simulink model "MOD_TC"  (R2012b)
settings: Solver=ode45  SolverMode=SingleTasking  StartTime=0.0  StopTime=10.0  RelTol=1e-3  AbsTol=1e-6
libraries: commanapbnd3 x4, simulink_extras x2, dsparch4 x1, commsynccomp2 x1
settings Model: ExtModeTrigMode=oneshot  ExtModeArmWhenConnect=off  Creator=Juan  LastModifiedBy=root
settings DataIOCC: LimitDataPoints=off  SignalLoggingSaveFormat=ModelDataLogs
settings OptimizationCC: BlockReduction=off  BooleanDataType=off
settings DebuggingCC: SaveWithParameterizedLinksMsg=none  SignalResolutionControl=TryResolveAllWithWarning  SolverPrmCheckMsg=none  MultiTaskDSMMsg=warning  MultiTaskCondExecSysMsg=none  FcnCallInpInsideContextMsg=UseLocalSettings  StrictBusMsg=None
settings HardwareCC: TargetUnknown=on
settings RTWCC: TemplateMakefile=grt_vc.tmf  IncludeERTFirstTime=on
settings CodeAppCC: CustomSymbolStrType=$N$R$M_T  InternalIdentifier=Shortened
settings GRTTargetCC: CombineOutputUpdateFcns=off  GRTInterface=on

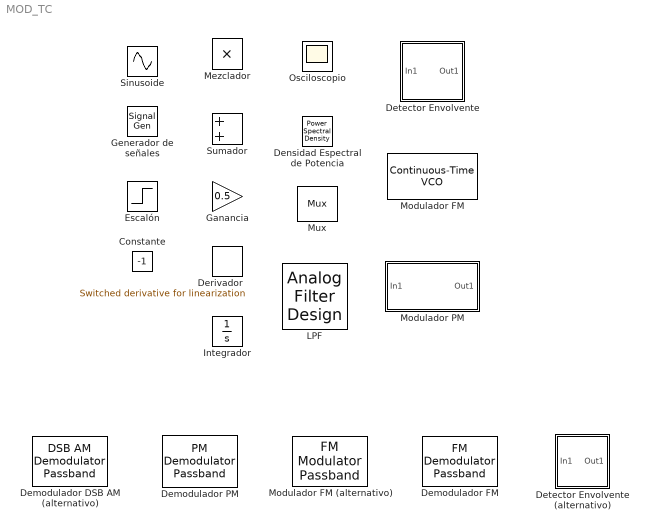
== system MOD_TC ==
  Constante : Constant  Value=-1
  Demodulador DSB AM (alternativo) : commanapbnd3/DSB AM Demodulator Passband  Fc=300  Ph=0  method=Butterworth  n=4  cf=300  Rp=0.1  Rs=50  Offset=1
  Demodulador FM : commanapbnd3/FM Demodulator Passband  Fc=300  Ph=0  Kc=50  Ho=100
  Demodulador PM : commanapbnd3/PM Demodulator Passband  Fc=300  Ph=0  Kc=pi/2  Ho=100
  Densidad Espectral de Potencia : simulink_extras/Additional Sinks/Power Spectral Density  npts=512  fftpts=512  HowOften=64  sampleT=0.1
  "Derivador " : simulink_extras/Linearization/Switched derivative for linearization  switchVal=0  derivConst=1000
  Detector Envolvente : Subsystem  mask(Envelope Detector (TELECO UPCT)){Tau=1}
      mask prompts: Tau "Tau (R*C) [sg]"
      mask help:
      | The Envelope Detector allows the demodulation of amplitude modulated signal which are not overmodulated.
      |
      | Select Tau (R*C) [s] with a value much higher than Tp (Carrier Period) and lower than Tm (Modulating Signal Period).
      |
      | E.g. If Tp=0.001 s, and Tm=10 s, then a suitable Tau could be between 0.1 and 1 s.
      mask Display: plot([0 0.0100 0.020 0.0301 0.0402 0.0502 0.06030 0.07035 0.08040 0.0904 0.1005 0.11055 0.1206 0.1306532 0.1407 0.15075 0.160804 0.17085 0.1809045 0.19095 0.2010 0.211055 0.2211 0.231155 0.24120 0.251256 0.26130 0.27135 0.28140703 0.291457 0.301507 0.3115 0.321608 0.331658 0.34170 0.35175 0.361809 0.371859 0.38190 0.39195 0.40201 0.412 0.422110552763819 0.432160804020101 0.442211055276382 0.452261306532663 0.462311557788945 0.472361809045226 0.482412060301508 0.492462311557789],[1.50000000000000 1.35725612705394 1.22809612961697 1.11122733102258 1.21161108958560 1.47509990887487 1.33472559289142 1.20770965925839 1.09278088982045 1.17321137879314 1.40287899306847 1.26937740590496 1.14858017447223 1.03927831947674 1.09864678512587 1.29052485666534 1.16771517921629 1.05659238776346 0.956044328060342 0.995576679540851 1.14920747660210 1.03984592591626 0.940891502761281 0.851353838010491 0.874697418425945 0.992951895818910 0.898460029646694 0.812960253434026 0.735596856683103 0.748707875672720 0.837224292404762 0.75755 0.68546 0.62023 0.63104 0.6973 0.6310 0.57096 0.51662 0.5345 0.5870 0.5312 0.48067 0.4349 0.4700 0.5170 0.4678 0.4233 0.3830 0.4454],[0 0.0100502512562814 0.0201005025125628 0.0301507537688442 0.0402010050251256 0.0502512562814070 0.0603015075376884 0.0703517587939699 0.0804020100502513 0.0904522613065327 0.100502512562814 0.110552763819095 0.120603015075377 0.130653266331658 0.140703517587940 0.150753768844221 0.160804020100503 0.170854271356784 0.180904522613065 0.190954773869347 0.201005025125628 0.211055276381910 0.221105527638191 0.231155778894472 0.241206030150754 0.251256281407035 0.261306532663317 0.271356783919598 0.281407035175879 0.291457286432161 0.301507537688442 0.311557788944724 0.321608040201005 0.331658291457286 0.341708542713568 0.351758793969849 0.361809045226131 0.371859296482412 0.381909547738693 0.391959798994975 0.402010050251256 0.412060301507538 0.422110552763819 0.432160804020101 0.442211055276382 0.452261306532663 0.462311557788945 0.472361809045226 0.482412060301508 0.492462311557789], [1.50000000000000 1.20993126439682 0.453301106657544 -0.474172583029756 -1.21161108958560 -1.47509990887487 -1.16831719880494 -0.418047916584565 0.478613777302988 1.17321137879314 1.40287899306847 1.09087247839569 0.371835504257245 -0.466298299188217 -1.09864678512587 -1.29052485666534 -0.985159188934220 -0.318978844871803 0.438787868134165 0.995576679540851 1.14920747660210 0.861359170684520 0.264132949337291 -0.399486171411829 -0.874697418425945 -0.992951895818910 -0.731189040830292 -0.211736977904714 0.353374570524558 0.748707875672720 0.837224292404762 0.606685035222284 0.165519860648553 -0.306548903245726 -0.631049231141791 -0.697375278761685 -0.498984597632528 -0.128122278411314 0.265600709413535 0.534545276542671 0.587098567823176 0.417229181498486 0.100873701918498 -0.236906206282143 -0.470081999110723 -0.517061222036970 -0.367697445635419 -0.0837430370887885 0.225899803116156 0.445463423116636])
  Detector Envolvente (alternativo) : Subsystem  RequirementInfo={} %GIDa_57ab6597_491d_46ba_9525_4d5ba1203f64  mask(Envelope Detector v2 (TELECO UPCT) (7 Marzo 2018)){Tau=0.2, Ts=0.001}
      mask prompts: Tau "Tiempo Descarga (Tau [s])"; Ts "Tiempo de Muestreo (Ts [s])"
      mask help:
      | The Envelope Detector allows the demodulation of amplitude modulated signal which are not overmodulated.
      |
      | Select Tau (R*C) [s] with a value much higher than Tp (Carrier Period) and lower than Tm (Modulating Signal Period).
      |
      | E.g. If Tp=0.001 s, and Tm=10 s, then a suitable Tau could be between 0.1 and 1 s.
      mask Display: plot([0 0.0100 0.020 0.0301 0.0402 0.0502 0.06030 0.07035 0.08040 0.0904 0.1005 0.11055 0.1206 0.1306532 0.1407 0.15075 0.160804 0.17085 0.1809045 0.19095 0.2010 0.211055 0.2211 0.231155 0.24120 0.251256 0.26130 0.27135 0.28140703 0.291457 0.301507 0.3115 0.321608 0.331658 0.34170 0.35175 0.361809 0.371859 0.38190 0.39195 0.40201 0.412 0.422110552763819 0.432160804020101 0.442211055276382 0.452261306532663 0.462311557788945 0.472361809045226 0.482412060301508 0.492462311557789],[1.50000000000000 1.35725612705394 1.22809612961697 1.11122733102258 1.21161108958560 1.47509990887487 1.33472559289142 1.20770965925839 1.09278088982045 1.17321137879314 1.40287899306847 1.26937740590496 1.14858017447223 1.03927831947674 1.09864678512587 1.29052485666534 1.16771517921629 1.05659238776346 0.956044328060342 0.995576679540851 1.14920747660210 1.03984592591626 0.940891502761281 0.851353838010491 0.874697418425945 0.992951895818910 0.898460029646694 0.812960253434026 0.735596856683103 0.748707875672720 0.837224292404762 0.75755 0.68546 0.62023 0.63104 0.6973 0.6310 0.57096 0.51662 0.5345 0.5870 0.5312 0.48067 0.4349 0.4700 0.5170 0.4678 0.4233 0.3830 0.4454],[0 0.0100502512562814 0.0201005025125628 0.0301507537688442 0.0402010050251256 0.0502512562814070 0.0603015075376884 0.0703517587939699 0.0804020100502513 0.0904522613065327 0.100502512562814 0.110552763819095 0.120603015075377 0.130653266331658 0.140703517587940 0.150753768844221 0.160804020100503 0.170854271356784 0.180904522613065 0.190954773869347 0.201005025125628 0.211055276381910 0.221105527638191 0.231155778894472 0.241206030150754 0.251256281407035 0.261306532663317 0.271356783919598 0.281407035175879 0.291457286432161 0.301507537688442 0.311557788944724 0.321608040201005 0.331658291457286 0.341708542713568 0.351758793969849 0.361809045226131 0.371859296482412 0.381909547738693 0.391959798994975 0.402010050251256 0.412060301507538 0.422110552763819 0.432160804020101 0.442211055276382 0.452261306532663 0.462311557788945 0.472361809045226 0.482412060301508 0.492462311557789], [1.50000000000000 1.20993126439682 0.453301106657544 -0.474172583029756 -1.21161108958560 -1.47509990887487 -1.16831719880494 -0.418047916584565 0.478613777302988 1.17321137879314 1.40287899306847 1.09087247839569 0.371835504257245 -0.466298299188217 -1.09864678512587 -1.29052485666534 -0.985159188934220 -0.318978844871803 0.438787868134165 0.995576679540851 1.14920747660210 0.861359170684520 0.264132949337291 -0.399486171411829 -0.874697418425945 -0.992951895818910 -0.731189040830292 -0.211736977904714 0.353374570524558 0.748707875672720 0.837224292404762 0.606685035222284 0.165519860648553 -0.306548903245726 -0.631049231141791 -0.697375278761685 -0.498984597632528 -0.128122278411314 0.265600709413535 0.534545276542671 0.587098567823176 0.417229181498486 0.100873701918498 -0.236906206282143 -0.470081999110723 -0.517061222036970 -0.367697445635419 -0.0837430370887885 0.225899803116156 0.445463423116636])
  Escalón : Step  Time=0
  Ganancia : Gain  Gain=0.5  SaturateOnIntegerOverflow=on  OutDataTypeStr=Inherit: Same as input  ParamDataTypeStr=Inherit: Same as input
  Generador de señales : SignalGenerator  Frequency=10  Units=rad/sec
  Integrador : Integrator
  LPF : dsparch4/Analog Filter Design  method=Butterworth  filttype=Lowpass  N=5  Wlo=2*2*pi  Whi=80  Rp=1  Rs=180
  Mezclador : Product  SaturateOnIntegerOverflow=on  RndMeth=Zero  InputSameDT=on  OutDataTypeStr=Inherit: Same as first input
  Modulador FM : commsynccomp2/Continuous-Time VCO  Ac=1  Fc=10  Kc=1  Ph=0
  Modulador FM (alternativo) : commanapbnd3/FM Modulator Passband  Fc=300  Ph=0  Kc=50
  Modulador PM : Subsystem  mask(Phase Modulator (PM) - Teleco UPCT){A=10, S=1, F=10, IP=0}
      mask prompts: A "Carrier_Amplitude"; S "Phase_Sensitivity (rad/V)"; F "Frequency_Carrier (Hz)"; IP "Initial_Phase (rad)"
      mask help:
      | Modulate the input signal using the phase modulation method.
      |
      | The input signal must be a scalar.
      mask Display:
      | plot(0,0,100,100,[4.5*[0:10]+5 50 50 50 50+4.5*[0:.15:10]],[10*sin([0:10]*pi/5)+85 85 99 75 85+10*[sin([0:.15:10]*pi*2+cumsum(sin([0:.15:10]*pi/5))/2)]]);
      | disp('PM - UPCT')
  Mux : Mux  Inputs=2
      settings: DisplayOption=signals
  Osciloscopio : Scope
      settings: TickLabels=on  YMin=-10  YMax=10
  Sinusoide : Sin  SampleTime=0
  "Sumador " : Sum  SaturateOnIntegerOverflow=on  InputSameDT=on  OutDataTypeStr=Inherit: Same as first input

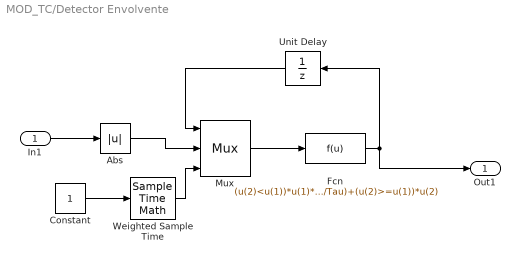
== system MOD_TC/Detector Envolvente ==
  In1 : Inport
  Abs : Abs
  Constant : Constant
  Fcn : Fcn  Expr=(u(2)<u(1))*u(1)*exp(-u(3)/Tau)+(u(2)>=u(1))*u(2)
  Mux : Mux  Inputs=3
      settings: DisplayOption=signals
  Unit Delay : UnitDelay  SampleTime=-1
  Weighted Sample Time : SampleTimeMath  TsampMathOp=Ts Only
  Out1 : Outport
  wires:
  Unit Delay/1 -> Mux/1
  Mux/1 -> Fcn/1
  Abs/1 -> Mux/2
  Fcn/1 -> Out1/1, Unit Delay/1
  In1/1 -> Abs/1
  Constant/1 -> Weighted Sample Time/1
  Weighted Sample Time/1 -> Mux/3

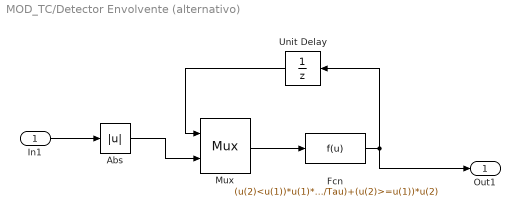
== system MOD_TC/Detector Envolvente (alternativo) ==
  In1 : Inport
  Abs : Abs
  Fcn : Fcn  Expr=(u(2)<u(1))*u(1)*exp(-Ts/Tau)+(u(2)>=u(1))*u(2)
  Mux : Mux  Inputs=2
      settings: DisplayOption=signals
  Unit Delay : UnitDelay  SampleTime=-1
  Out1 : Outport
  wires:
  In1/1 -> Abs/1
  Fcn/1 -> Unit Delay/1, Out1/1
  Abs/1 -> Mux/2
  Mux/1 -> Fcn/1
  Unit Delay/1 -> Mux/1

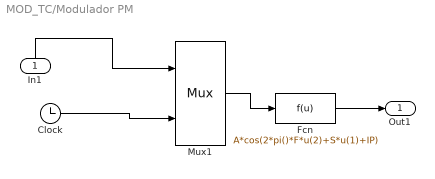
== system MOD_TC/Modulador PM ==
  In1 : Inport
  Clock : Clock
  Fcn : Fcn  Expr=A*cos(2*pi()*F*u(2)+S*u(1)+IP)
  Mux1 : Mux  Inputs=2
      settings: DisplayOption=signals
  Out1 : Outport
  wires:
  Clock/1 -> Mux1/2
  Mux1/1 -> Fcn/1
  In1/1 -> Mux1/1
  Fcn/1 -> Out1/1
